simulink model "M5HatJoy_BLE23a"  (R2023a)
settings: Solver=FixedStepAuto  StartTime=0.0  StopTime=Inf  FixedStep=1/50  RelTol=1e-3  EnableMultiTasking=on
settings Model: ExtModeTrigDuration=2  Creator=totani  LastModifiedBy=totani
settings SolverCC: AutoInsertRateTranBlk=on
settings DataIOCC: SaveOutput=off  DSMLogging=off  SaveTime=off  ReturnWorkspaceOutputs=off
settings OptimizationCC: EnhancedBackFolding=on  PassReuseOutputArgsAs=Individual arguments  ZeroExternalMemoryAtStartup=off  ZeroInternalMemoryAtStartup=off  MaxStackSize=64  OptimizeBlockOrder=speed  DifferentSizesBufferReuse=on  OptimizationCustomize=off  EfficientTunableParamExpr=on
settings DebuggingCC: ParameterTunabilityLossMsg=error
settings HardwareCC: ProdBitPerPointer=32  ProdBitPerSizeT=32  ProdBitPerPtrDiffT=32  ProdLargestAtomicInteger=Long  ProdLargestAtomicFloat=Double  ProdWordSize=32  ProdHWDeviceType=ARM Compatible->ARM Cortex  UseEmbeddedCoderFeatures=off  UseSimulinkCoderFeatures=off
settings SFSimCC: MATLABDynamicMemAlloc=off
settings RTWCC: Description=Embedded Coder  SystemTargetFile=ert.tlc  HardwareBoard=ESP32-WROOM(Arduino Compatible)  TLCOptions="-aInlineSetEventsForThisBaseRateFcn=TLC_FALSE -aSuppressMultiTaskScheduler=TLC_FALSE  -aRateBasedStepFcn=0"  TemplateMakefile=ert_default_tmf  Toolchain=ESP32  BuildConfiguration=Faster Runs  GPUComputeCapability=5.0
settings CodeAppCC: ForceParamTrailComments=on  IgnoreCustomStorageClasses=off  OperatorAnnotations=on  SimulinkDataObjDesc=on  SFDataObjDesc=on  InsertBlockDesc=on
settings ERTTargetCC: SupportContinuousTime=on  SupportNonInlinedSFcns=on  SupportVariableSizeSignals=on  ExtModeTransport=3  ExtModeStaticAlloc=on  ExtModeAutomaticAllocSize=off  ExtModeStaticAllocSize=65536  ExtModeMexFile=ext_xcp  ExtModeIntrfLevel=Level2 - Open

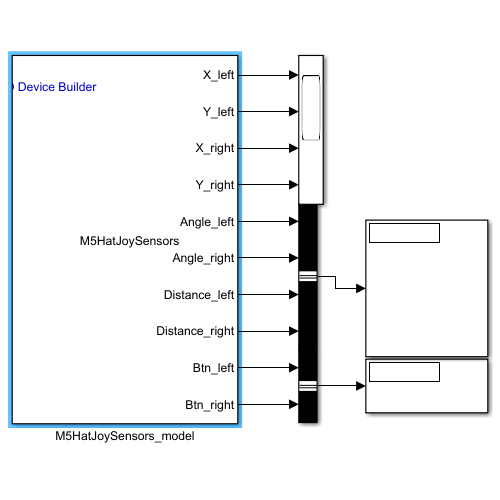
[thumbnail: Simulink's stored preview of the top-level diagram]
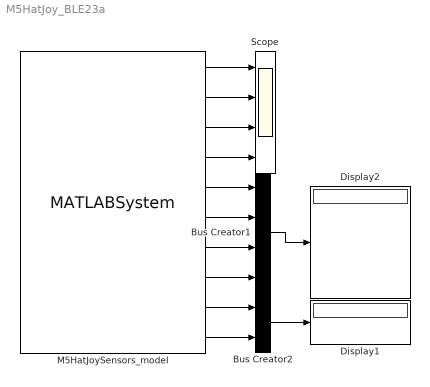
== system M5HatJoy_BLE23a ==
  Bus Creator1 : BusCreator  Inputs=4
  Bus Creator2 : BusCreator  Inputs=2
  Display1 : Display
  Display2 : Display
  M5HatJoySensors_model : MATLABSystem  System=M5HatJoySensors  LED_Color=0x55FF00  SampleTime=-1
      mask Type: M5HatJoySensors
      mask Display:
      | color('white');plot([100,100,100,100]*1,[100,100,100,100]*1);plot([100,100,100,100]*0,[100,100,100,100]*0);color('blue');text(38, 92, 'IO Device Builder','horizontalAlignment', 'right');
      | color('black');text(52,50,' M5HatJoySensors','horizontalAlignment','center');
      | port_label('output',1,'X_left');port_label('output',2,'Y_left');port_label('output',3,'X_right');port_label('output',4,'Y_right');port_label('output',5,'Angle_left');port_label('output',6,'Angle_right');port_label('output',7,'Distance_left');port_label('output',8,'Distance_right');port_label('output',9,'Btn_left');port_label('output',10,'Btn_right');
  Scope : Scope  NumInputPorts=4
  wires:
  M5HatJoySensors_model/1 -> Scope/1
  M5HatJoySensors_model/2 -> Scope/2
  M5HatJoySensors_model/3 -> Scope/3
  M5HatJoySensors_model/4 -> Scope/4
  M5HatJoySensors_model/5 -> Bus Creator1/1
  M5HatJoySensors_model/6 -> Bus Creator1/2
  M5HatJoySensors_model/7 -> Bus Creator1/3
  M5HatJoySensors_model/8 -> Bus Creator1/4
  M5HatJoySensors_model/9 -> Bus Creator2/1
  M5HatJoySensors_model/10 -> Bus Creator2/2
  Bus Creator2/1 -> Display1/1
  Bus Creator1/1 -> Display2/1
